simulink model "ModelTeachingFactory"  (R2020b)
settings: Solver=VariableStepAuto  StartTime=0.0  StopTime=10.0  RelTol=1e-3
settings Model: Creator=kaebi  LastModifiedBy=kaebi

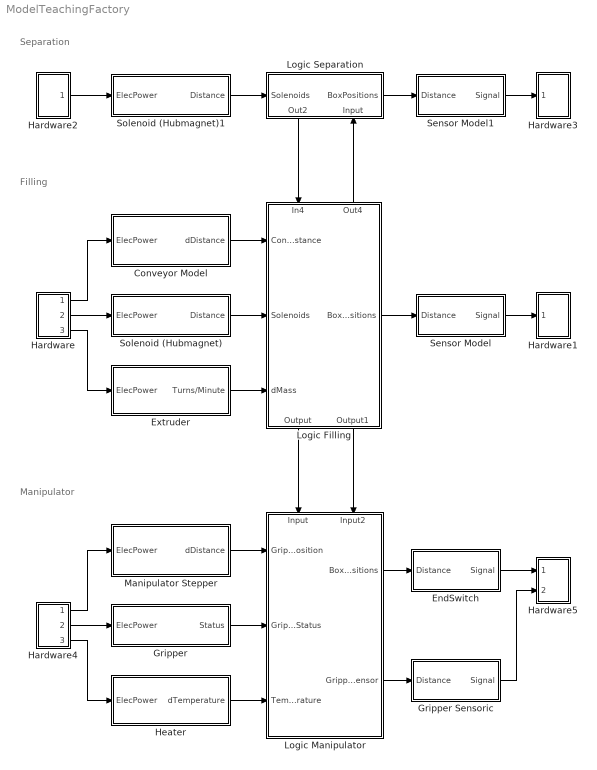
== system ModelTeachingFactory ==
  note: Filling
  note: Separation
  note: Manipulator
  Conveyor Model : Subsystem
  EndSwitch : Subsystem
  Extruder : Subsystem
  Gripper : Subsystem
  Gripper Sensoric : Subsystem
  Hardware : Subsystem
  Hardware1 : Subsystem
  Hardware2 : Subsystem
  Hardware3 : Subsystem
  Hardware4 : Subsystem
  Hardware5 : Subsystem
  Heater : Subsystem
  Logic Filling : Subsystem
      settings: PortSchema="{\"entries\":[{\"content\":{\"sides\":[{\"content\":{\"connectorIds\":[\"In1\",\"In2\",\"In3\"]},\"type\":\"ConnectorPlacement.EquallySpacedRectSide\",\"uuid\":\"607da6d4-7d9a-49ad-8c47-e0b53e85162d\"},{\"content\":{\"connectorIds\":[\"Out1\"],\"side\":\"RIGHT\"},\"type\":\"ConnectorPlacement.EquallySpacedRectSide\",\"uuid\":\"7fb4784c-1535-463a-bff7-b2e5cd5ee292\"},{\"content\":{\"connectorIds\":[\"In4\",\"Out4\"],\"side\":\"TOP\"},\"type\":\"ConnectorPlacement.EquallySpacedRectSide\",\"uuid\":\"a7a131b6-49eb-49b1-86b7-c2fc797e86d2\"},{\"content\":{\"connectorIds\":[\"Out2\",\"Out3\"],\"side\":\"BOTTOM\"},\"type\":\"ConnectorPlacement.EquallySpacedRectSide\",\"uuid\":\"12ae16ca-fefc-4806-b133-6ced7321f41b\"},{\"content\":{\"connectorIds\":[],\"side\":\"HIDDEN\"},\"type\":\"ConnectorPlacement.EquallySpacedRectSide\",\"uuid\":\"292e56e1-0c3f-42c5-979f-4bd531eb655e\"}]},\"type\":\"ConnectorPlacement.EquallySpacedConnector\",\"uuid\":\"2a1cf29e-3981-4c3c-849c-eb5a91e5efbf\"}],\"packageUris\":[\"http://schema.mathworks.com/mf0/Connector/R2020b\"],\"version\":\"1.0\"}"
  Logic Manipulator : Subsystem
      settings: PortSchema="{\"entries\":[{\"content\":{\"sides\":[{\"content\":{\"connectorIds\":[\"In1\",\"In2\",\"In3\"]},\"type\":\"ConnectorPlacement.EquallySpacedRectSide\",\"uuid\":\"607da6d4-7d9a-49ad-8c47-e0b53e85162d\"},{\"content\":{\"connectorIds\":[\"Out1\",\"Out2\"],\"side\":\"RIGHT\"},\"type\":\"ConnectorPlacement.EquallySpacedRectSide\",\"uuid\":\"7fb4784c-1535-463a-bff7-b2e5cd5ee292\"},{\"content\":{\"connectorIds\":[\"In4\",\"In5\"],\"side\":\"TOP\"},\"type\":\"ConnectorPlacement.EquallySpacedRectSide\",\"uuid\":\"a7a131b6-49eb-49b1-86b7-c2fc797e86d2\"},{\"content\":{\"connectorIds\":[],\"side\":\"HIDDEN\"},\"type\":\"ConnectorPlacement.EquallySpacedRectSide\",\"uuid\":\"292e56e1-0c3f-42c5-979f-4bd531eb655e\"}]},\"type\":\"ConnectorPlacement.EquallySpacedConnector\",\"uuid\":\"2a1cf29e-3981-4c3c-849c-eb5a91e5efbf\"}],\"packageUris\":[\"http://schema.mathworks.com/mf0/Connector/R2020b\"],\"version\":\"1.0\"}"
  Logic Separation : Subsystem
      settings: PortSchema="{\"entries\":[{\"content\":{\"sides\":[{\"content\":{\"connectorIds\":[\"In1\"]},\"type\":\"ConnectorPlacement.EquallySpacedRectSide\",\"uuid\":\"d6ecdedd-6b8f-4d80-89f5-c8b517abd7c3\"},{\"content\":{\"connectorIds\":[\"Out1\"],\"side\":\"RIGHT\"},\"type\":\"ConnectorPlacement.EquallySpacedRectSide\",\"uuid\":\"8e821b71-510e-4448-ae8c-3c65ed8f18d7\"},{\"content\":{\"connectorIds\":[],\"side\":\"TOP\"},\"type\":\"ConnectorPlacement.EquallySpacedRectSide\",\"uuid\":\"2248ac2e-2b7d-4162-bb55-419838faa2ef\"},{\"content\":{\"connectorIds\":[\"Out2\",\"In2\"],\"side\":\"BOTTOM\"},\"type\":\"ConnectorPlacement.EquallySpacedRectSide\",\"uuid\":\"4363741d-a4d8-4dd1-87d3-b20b93c27d83\"},{\"content\":{\"connectorIds\":[],\"side\":\"HIDDEN\"},\"type\":\"ConnectorPlacement.EquallySpacedRectSide\",\"uuid\":\"323a68a2-e1fd-42e7-8320-8e1664bce830\"}]},\"type\":\"ConnectorPlacement.EquallySpacedConnector\",\"uuid\":\"d6ff5951-2e4c-46b6-8339-6c4251d1a79f\"}],\"packageUris\":[\"http://schema.mathworks.com/mf0/Connector/R2020b\"],\"version\":\"1.0\"}"
  Manipulator Stepper : Subsystem
  Sensor Model : Subsystem
  Sensor Model1 : Subsystem
  Solenoid (Hubmagnet) : Subsystem
  Solenoid (Hubmagnet)1 : Subsystem
  wires:
  Solenoid (Hubmagnet)/1(Distance) -> Logic Filling/2(Solenoids)
  Conveyor Model/1(dDistance) -> Logic Filling/1(ConvDistance)
  Logic Filling/1(BoxPositions) -> Sensor Model/1(Distance)
  Sensor Model/1(Signal) -> Hardware1/1(Input)
  Hardware/1(Out1) -> Conveyor Model/1(ElecPower)
  Hardware/2(Out2) -> Solenoid (Hubmagnet)/1(ElecPower)
  Hardware/3(Out3) -> Extruder/1(ElecPower)
  Extruder/1(Turns/Minute) -> Logic Filling/3(dMass)
  Sensor Model1/1(Signal) -> Hardware3/1(Input)
  Logic Separation/1(BoxPositions) -> Sensor Model1/1(Distance)
  Solenoid (Hubmagnet)1/1(Distance) -> Logic Separation/1(Solenoids)
  Hardware2/1(Output) -> Solenoid (Hubmagnet)1/1(ElecPower)
  Logic Separation/2(Out2) -> Logic Filling/4(In4)
  Heater/1(dTemperature) -> Logic Manipulator/3(Temperature)
  Hardware4/3(Out3) -> Heater/1(ElecPower)
  Hardware4/2(Out2) -> Gripper/1(ElecPower)
  Hardware4/1(Out1) -> Manipulator Stepper/1(ElecPower)
  EndSwitch/1(Signal) -> Hardware5/1(Input)
  Logic Manipulator/1(BoxPositions) -> EndSwitch/1(Distance)
  Manipulator Stepper/1(dDistance) -> Logic Manipulator/1(GripperPosition)
  Gripper/1(Status) -> Logic Manipulator/2(GripperStatus)
  Logic Filling/2(Output) -> Logic Manipulator/4(Input)
  Logic Manipulator/2(GripperSensor) -> Gripper Sensoric/1(Distance)
  Gripper Sensoric/1(Signal) -> Hardware5/2(Input2)
  Logic Filling/4(Out4) -> Logic Separation/2(Input)
  Logic Filling/3(Output1) -> Logic Manipulator/5(Input2)

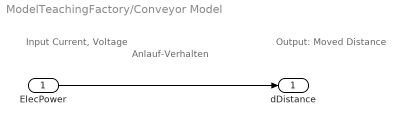
== system ModelTeachingFactory/Conveyor Model ==
  note: Input
      | Current, Voltage
  note: Anlauf-Verhalten
  note: Output:
      | Moved Distance
  ElecPower : Inport
  dDistance : Outport
  wires:
  ElecPower/1 -> dDistance/1

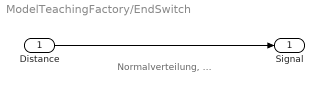
== system ModelTeachingFactory/EndSwitch ==
  note: Normalverteilung, ...
  Distance : Inport
  Signal : Outport
  wires:
  Distance/1 -> Signal/1

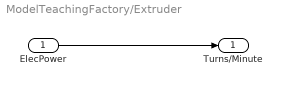
== system ModelTeachingFactory/Extruder ==
  ElecPower : Inport
  Turns/Minute : Outport
  wires:
  ElecPower/1 -> Turns/Minute/1

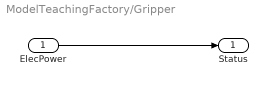
== system ModelTeachingFactory/Gripper ==
  ElecPower : Inport
  Status : Outport
  wires:
  ElecPower/1 -> Status/1

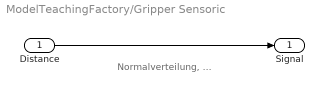
== system ModelTeachingFactory/Gripper Sensoric ==
  note: Normalverteilung, ...
  Distance : Inport
  Signal : Outport
  wires:
  Distance/1 -> Signal/1

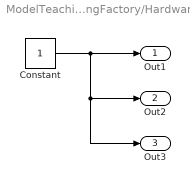
== system ModelTeachingFactory/Hardware ==
  Constant : Constant
  Out1 : Outport
  Out2 : Outport  Port=2
  Out3 : Outport  Port=3
  wires:
  Constant/1 -> Out1/1, Out3/1, Out2/1

== system ModelTeachingFactory/Hardware1 ==
  Input : Inport

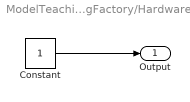
== system ModelTeachingFactory/Hardware2 ==
  Constant : Constant
  Output : Outport
  wires:
  Constant/1 -> Output/1

== system ModelTeachingFactory/Hardware3 ==
  Input : Inport

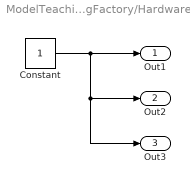
== system ModelTeachingFactory/Hardware4 ==
  Constant : Constant
  Out1 : Outport
  Out2 : Outport  Port=2
  Out3 : Outport  Port=3
  wires:
  Constant/1 -> Out2/1, Out3/1, Out1/1

== system ModelTeachingFactory/Hardware5 ==
  Input : Inport
  Input2 : Inport  Port=2

== system ModelTeachingFactory/Heater ==
  ElecPower : Inport
  dTemperature : Outport
  wires:
  ElecPower/1 -> dTemperature/1

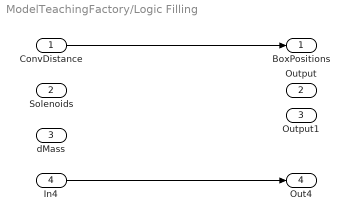
== system ModelTeachingFactory/Logic Filling ==
  ConvDistance : Inport
  Solenoids : Inport  Port=2
  dMass : Inport  Port=3
  In4 : Inport  Port=4
  BoxPositions : Outport
  Output : Outport  Port=2
  Output1 : Outport  Port=3
  Out4 : Outport  Port=4
  wires:
  ConvDistance/1 -> BoxPositions/1
  In4/1 -> Out4/1

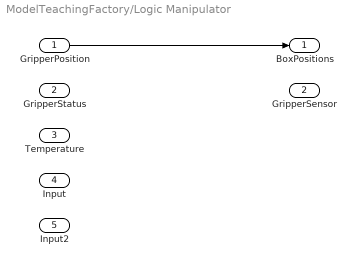
== system ModelTeachingFactory/Logic Manipulator ==
  GripperPosition : Inport
  GripperStatus : Inport  Port=2
  Temperature : Inport  Port=3
  Input : Inport  Port=4
  Input2 : Inport  Port=5
  BoxPositions : Outport
  GripperSensor : Outport  Port=2
  wires:
  GripperPosition/1 -> BoxPositions/1

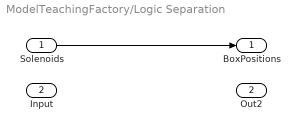
== system ModelTeachingFactory/Logic Separation ==
  Solenoids : Inport
  Input : Inport  Port=2
  BoxPositions : Outport
  Out2 : Outport  Port=2
  wires:
  Solenoids/1 -> BoxPositions/1

== system ModelTeachingFactory/Manipulator Stepper ==
  note: Output:
      | Moved Distance
  note: Anlauf-Verhalten
  note: Input
      | Current, Voltage
  ElecPower : Inport
  dDistance : Outport
  wires:
  ElecPower/1 -> dDistance/1

== system ModelTeachingFactory/Sensor Model ==
  note: Normalverteilung, ...
  Distance : Inport
  Signal : Outport
  wires:
  Distance/1 -> Signal/1

== system ModelTeachingFactory/Sensor Model1 ==
  note: Normalverteilung, ...
  Distance : Inport
  Signal : Outport
  wires:
  Distance/1 -> Signal/1

== system ModelTeachingFactory/Solenoid (Hubmagnet) ==
  ElecPower : Inport
  Distance : Outport
  wires:
  ElecPower/1 -> Distance/1

== system ModelTeachingFactory/Solenoid (Hubmagnet)1 ==
  ElecPower : Inport
  Distance : Outport
  wires:
  ElecPower/1 -> Distance/1
